simulink model "Vehicle_Model_999_Modular"  (R2025b)
settings: Solver=ode23tb  StartTime=0.0  StopTime=20  MaxStep=0.001  RelTol=1e-3
values from neighbouring files (symbols this model uses):
  aero_par = struct()    [Load_aero_parameters.m]
  init_r = 0    [Run_this_first.m]
  init_vx = 0    [Run_this_first.m]
  init_vy = 0    [Run_this_first.m]
  m = Par.m    [LapSim_Endurance_final_ts_v2.m]    (also in Lap_Sim_Final_inverse.m = Par.Mass; Lapsim_Endurance_final_ts.m; New_LapSim_final_ts_v1.m = Par.Mass; Torque_vectoring_lookup_table_v3.m = 270)
  Par = struct()    [Load_vehicle_parameters.m]
  sus_par = struct()    [Load_sus_parameters.m]
  TireData = []    [Lapsim_final_for_app.m]
  V_ref = 45    [Run_this_first.m]
undefined symbols (not defined in the file or in its folder): Battery, Brake_Val, HP, Ki_data, Kp_data, Motor, steer_input, Steer_Val, Throttle_Val, vx_breakpoints
libraries: simulink x7, autolibshared x2, BatteryEstimators x1, simulink_extras x1
(part 2 of 3)

== system Vehicle_Model_999_Modular/Vehicle dynamics/Fx, Fy calculations/Slip_angle_calculation ==
  Bus Selector25 : BusSelector  OutputSignals=Longitudinal_vel
  Bus Selector26 : BusSelector  OutputSignals=Lateral_vel
  Bus Selector27 : BusSelector  OutputSignals=Yaw_rate
  Bus Selector28 : BusSelector  OutputSignals=Steer_FL
  Bus Selector29 : BusSelector  OutputSignals=Steer_FR
  Slip Angles : MATLAB Function  TreatAsAtomicUnit=on
  Subsystem : Subsystem
  Visualize Slip_angle : Subsystem
  effective_slip_angle : Outport
  wires:
  Bus Selector26/1 -> Slip Angles/2(Lateral_vel)  "<Lateral_vel>"
  Bus Selector27/1 -> Slip Angles/3(yawrate)  "<Yaw_rate>"
  [Steer_bus] -> Bus Selector29/1, Bus Selector28/1
  [chassisbus] -> Bus Selector27/1, Bus Selector26/1, Bus Selector25/1
  Bus Selector25/1 -> Slip Angles/1(Longitudinal_vel)  "<Longitudinal_vel>"
  Slip Angles/1(slip_angles) -> Subsystem/2(slip_angles)
  Bus Selector28/1 -> Slip Angles/4(Steer_FL)  "<Steer_FL>"
  Bus Selector29/1 -> Slip Angles/5(Steer_FR)  "<Steer_FR>"
  Subsystem/1(slip_ratio) -> Visualize Slip_angle/1(slip_angle), effective_slip_angle/1  "effective_slip_angle"
  [Toe_angle] -> Subsystem/1(toe)

== system Vehicle_Model_999_Modular/Vehicle dynamics/Fx, Fy calculations/Slip_ratio_calculation ==
  Bus Selector21 : BusSelector  OutputSignals=Longitudinal_vel
  Bus Selector22 : BusSelector  OutputSignals=Yaw_rate
  Bus Selector23 : BusSelector  OutputSignals=Omega
  Bus Selector24 : BusSelector  OutputSignals=Lateral_vel
  Bus Selector32 : BusSelector  OutputSignals=Steer_FL
  Bus Selector33 : BusSelector  OutputSignals=Steer_FR
  Visualize Slip_ratios : Subsystem  Commented=on
  slip ratios : MATLAB Function  TreatAsAtomicUnit=on
  slip_ratios : Outport
  wires:
  [Steer_bus] -> Bus Selector32/1, Bus Selector33/1
  Bus Selector21/1 -> slip ratios/1(Vx)  "<Longitudinal_vel>"
  Bus Selector23/1 -> slip ratios/4(Omega)  "<Omega>"
  Bus Selector32/1 -> slip ratios/5(Steer_FL)  "<Steer_FL>"
  [chassisbus] -> Bus Selector22/1, Bus Selector24/1, Bus Selector21/1
  Bus Selector22/1 -> slip ratios/3(yawrate)  "<Yaw_rate>"
  Bus Selector33/1 -> slip ratios/6(Steer_FR)  "<Steer_FR>"
  Bus Selector24/1 -> slip ratios/2(Vy)  "<Lateral_vel>"
  [Wheel_bus] -> Bus Selector23/1
  slip ratios/1(slip_ratios) -> Visualize Slip_ratios/1(slip_ratio), slip_ratios/1  "slip_ratios"

== system Vehicle_Model_999_Modular/Vehicle dynamics/Fx, Fy calculations/Tyre_relaxation ==
  Fx_ss : Inport
  Bus Selector : BusSelector  OutputSignals=Longitudinal_vel
  Integrator : Integrator
  MATLAB Function : MATLAB Function  TreatAsAtomicUnit=on
  Fx_w : Outport
  wires:
  Fx_ss/1 -> MATLAB Function/1(Fx_ss)
  MATLAB Function/1(Fx_dot) -> Integrator/1
  Integrator/1 -> Fx_w/1, MATLAB Function/2(Fx_act)
  Bus Selector/1 -> MATLAB Function/3(Vx)  "<Longitudinal_vel>"
  [chassisbus] -> Bus Selector/1

== system Vehicle_Model_999_Modular/Vehicle dynamics/Fx, Fy calculations/Visualise_Fy_B ==
  Fy_B : Inport
  MATLAB Function : MATLAB Function  TreatAsAtomicUnit=on
  Visualise Fy_B : Scope  Commented=on  NumInputPorts=4
  wires:
  Fy_B/1 -> MATLAB Function/1(Fy_tire)
  MATLAB Function/2(Fy_B_fr) -> Visualise Fy_B/2  "Fy_B_fr"
  MATLAB Function/4(Fy_B_rr) -> Visualise Fy_B/4  "Fy_B_rr"
  MATLAB Function/1(Fy_B_fl) -> Visualise Fy_B/1  "Fy_B_fl"
  MATLAB Function/3(Fy_B_rl) -> Visualise Fy_B/3  "Fy_B_rl"

== system Vehicle_Model_999_Modular/Vehicle dynamics/Fx, Fy calculations/Visualiser ==
  mz : Inport
  mu_x : Inport  Port=2
  mu_y : Inport  Port=3
  Demux : Demux
  Demux1 : Demux
  Demux2 : Demux
  Scope : Scope  NumInputPorts=4
  Scope1 : Scope  NumInputPorts=4
  Scope2 : Scope  NumInputPorts=4
  wires:
  mz/1 -> Demux/1
  Demux/1 -> Scope/1
  Demux/2 -> Scope/2
  Demux/3 -> Scope/3
  Demux/4 -> Scope/4
  Demux1/3 -> Scope1/3
  Demux1/2 -> Scope1/2
  mu_x/1 -> Demux1/1
  Demux1/1 -> Scope1/1
  Demux1/4 -> Scope1/4
  Demux2/3 -> Scope2/3
  Demux2/2 -> Scope2/2
  mu_y/1 -> Demux2/1
  Demux2/1 -> Scope2/1
  Demux2/4 -> Scope2/4

== system Vehicle_Model_999_Modular/Vehicle dynamics/Steering/Steering Kinematics ==
  Steer_Input : Inport
  Ackermann_Pct : Inport  Port=2
  Bus Creator1 : BusCreator  Inputs=2
  Steering Kinematics : MATLAB Function  TreatAsAtomicUnit=on
  To Workspace : ToWorkspace  VariableName=steer_L  SaveFormat=Timeseries  SampleTime=-1
  To Workspace1 : ToWorkspace  VariableName=steer_R  SaveFormat=Timeseries  SampleTime=-1
  Steering Angles : Outport
  wires:
  Steering Kinematics/1(Steer_FL) -> Bus Creator1/1, To Workspace/1  "Steer_FL"
  Steer_Input/1 -> Steering Kinematics/1(Steer_Input)
  Steering Kinematics/2(Steer_FR) -> Bus Creator1/2, To Workspace1/1  "Steer_FR"
  Ackermann_Pct/1 -> Steering Kinematics/2(Ackermann_Pct)
  Bus Creator1/1 -> Steering Angles/1

== system Vehicle_Model_999_Modular/Vehicle dynamics/Suspension/Camber ==
  Zs_static : Inport
  Zs : Inport  Port=2
  DynamicCamber_FromHP_Zmeters : MATLAB Function  TreatAsAtomicUnit=on
  Subsystem : Subsystem
  Subsystem1 : Subsystem  Commented=on
  Subsystem2 : Subsystem  Commented=on
  camber_angle : Outport
  wires:
  DynamicCamber_FromHP_Zmeters/1(Camber) -> camber_angle/1, Subsystem/1(Camber)
  Zs/1 -> DynamicCamber_FromHP_Zmeters/1(Zs)
  Zs_static/1 -> DynamicCamber_FromHP_Zmeters/2(Zs_static)
  DynamicCamber_FromHP_Zmeters/2(dynamic_camber_visualisation) -> Subsystem1/1(dynamic_camber)
  DynamicCamber_FromHP_Zmeters/3(static_camber_visualisation) -> Subsystem2/1(static_camber)

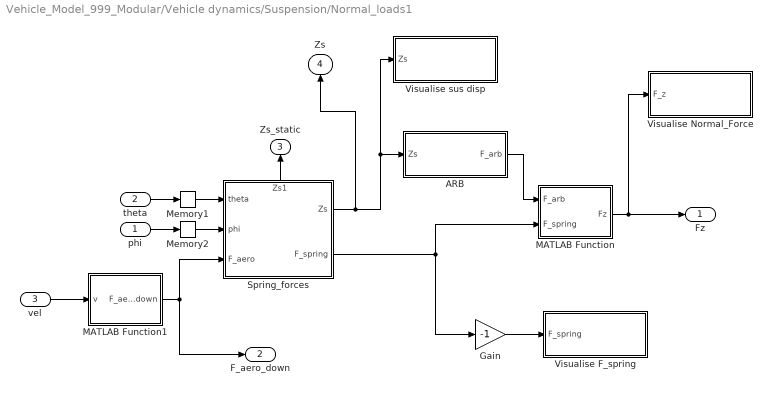
== system Vehicle_Model_999_Modular/Vehicle dynamics/Suspension/Normal_loads1 ==
  phi : Inport
  theta : Inport  Port=2
  vel : Inport  Port=3
  ARB : Subsystem
  Gain : Gain  Gain=-1
  MATLAB Function : MATLAB Function  TreatAsAtomicUnit=on
  MATLAB Function1 : MATLAB Function  TreatAsAtomicUnit=on
  Memory1 : Memory
  Memory2 : Memory
  Spring_forces : Subsystem
      settings: PortSchema="{\"entries\":[{\"content\":{\"sides\":[{\"content\":{\"connectorIds\":[\"In1\",\"In2\",\"In3\"]},\"type\":\"ConnectorPlacement.EquallySpacedRectSide\",\"uuid\":\"355bde33-3e3d-4de3-a05a-1287e2d3eebd\"},{\"content\":{\"connectorIds\":[\"Out1\",\"Out2\"],\"side\":\"RIGHT\"},\"type\":\"ConnectorPlacement.EquallySpacedRectSide\",\"uuid\":\"644c8213-6936-480f-b4bc-76ae135da058\"},{\"content\":{\"connectorIds\":[\"Out3\"],\"side\":\"TOP\"},\"type\":\"ConnectorPlacement.EquallySpacedRectSide\",\"uuid\":\"02c95e6b-ea4d-4952-978a-25b4914c2c12\"}]},\"type\":\"ConnectorPlacement.EquallySpacedConnector\",\"uuid\":\"3ff29f82-1f4c-432e-8c89-df3d4bc3a019\"}],\"packageUris\":[\"http://schema.mathworks.com/mf0/Connector/R2020b\"],\"version\":\"1.0\"}"
  Visualise F_spring : Subsystem
  Visualise Normal_Force : Subsystem
  Visualise sus disp : Subsystem
  Fz : Outport
  F_aero_down : Outport  Port=2
  Zs_static : Outport  Port=3
  Zs : Outport  Port=4
  wires:
  theta/1 -> Memory1/1
  phi/1 -> Memory2/1
  ARB/1(F_arb) -> MATLAB Function/1(F_arb)
  MATLAB Function/1(Fz) -> Visualise Normal_Force/1(F_z), Fz/1
  vel/1 -> MATLAB Function1/1(v)
  MATLAB Function1/1(F_aero_down) -> F_aero_down/1, Spring_forces/3(F_aero)
  Spring_forces/2(F_spring) -> MATLAB Function/2(F_spring), Gain/1
  Spring_forces/1(Zs) -> Visualise sus disp/1(Zs), ARB/1(Zs), Zs/1
  Spring_forces/3(Zs1) -> Zs_static/1
  Memory1/1 -> Spring_forces/1(theta)
  Memory2/1 -> Spring_forces/2(phi)
  Gain/1 -> Visualise F_spring/1(F_spring)

== system Vehicle_Model_999_Modular/Vehicle dynamics/Suspension/Toe_calculation ==
  Fy : Inport
  Fx : Inport  Port=2
  Mz : Inport  Port=3
  Mux1 : Mux
  toe_fl1 : MATLAB Function  TreatAsAtomicUnit=on
  Out2 : Outport
  wires:
  Mux1/1 -> Out2/1
  Mz/1 -> toe_fl1/3(Mz)
  Fx/1 -> toe_fl1/2(Fx_tire)
  Fy/1 -> toe_fl1/1(Fy_tire)
  toe_fl1/1(Toe_fl) -> Mux1/1
  toe_fl1/2(Toe_fr) -> Mux1/2
  toe_fl1/3(Toe_rl) -> Mux1/3
  toe_fl1/4(Toe_rr) -> Mux1/4

== system Vehicle_Model_999_Modular/Vehicle dynamics/Suspension/roll and pitch angles1 ==
  ax : Inport
  ay : Inport  Port=2
  F_aero : Inport  Port=3
  Phi_constants : MATLAB Function  TreatAsAtomicUnit=on
  Pitch : Subsystem
  Roll : Subsystem
  Scope : Scope  NumInputPorts=2
      settings: ActiveDisplayYMinimum=-1  ActiveDisplayYMaximum=1
  theta_constants : MATLAB Function  TreatAsAtomicUnit=on
  phi : Outport
  Theta : Outport  Port=2
  wires:
  ax/1 -> Pitch/3(ax)
  Phi_constants/1(K_phi) -> Roll/1(K_phi)
  Phi_constants/2(C_phi) -> Roll/2(C_phi)
  ay/1 -> Roll/3(ay)
  Roll/1(phi) -> phi/1, Scope/2
  Pitch/1(Theta) -> Scope/1, Theta/1
  theta_constants/1(K_theta) -> Pitch/1(K_theta)
  theta_constants/2(C_theta) -> Pitch/2(C_theta)
  F_aero/1 -> Pitch/4(downforce)

== system Vehicle_Model_999_Modular/Vehicle dynamics/Wheel_dynamics/Wheel Dynamics ==
  Fx_rr : Inport
  Bus Selector8 : BusSelector  OutputSignals=Fx_tyre
  Integrator : Integrator  InitialCondition=init_vx/Par.R0  LimitOutput=on  UpperSaturationLimit=1e6
  MATLAB Function : MATLAB Function  TreatAsAtomicUnit=on
  Scope : Scope
      settings: ActiveDisplayYMinimum=-1  ActiveDisplayYMaximum=1  DataLoggingVariableName=ScopeData3
  Omega : Outport
  wires:
  [Torque_inputs] -> MATLAB Function/1(T_in)
  Fx_rr/1 -> MATLAB Function/2(Fx_rr)
  MATLAB Function/1(Omega_dot) -> Integrator/1
  [Force_bus] -> Bus Selector8/1
  Bus Selector8/1 -> MATLAB Function/3(Fx_tire)  "<Fx_tyre>"
  Integrator/1 -> Scope/1, Omega/1, MATLAB Function/4(Omega)

== system Vehicle_Model_999_Modular/E-powertrain/Torque Distribution/Torque Vectoring/Target yaw rate ==
  steering angle : Inport
  Fz_4x1 : Inport  Port=2
  Dy : Inport  Port=3
  vx : Inport  Port=4
  MATLAB Function : MATLAB Function  TreatAsAtomicUnit=on
  target yaw rate : Outport
  ideal_yaw : Outport  Port=2
  wires:
  vx/1 -> MATLAB Function/1(vx)
  Fz_4x1/1 -> MATLAB Function/4(Fz)
  Dy/1 -> MATLAB Function/3(Dy)
  steering angle/1 -> MATLAB Function/2(delta)
  MATLAB Function/1(target_yaw) -> target yaw rate/1
  MATLAB Function/2(ideal_yaw) -> ideal_yaw/1

== system Vehicle_Model_999_Modular/Inputs/Brake_input_selector/Brake Variant Subsystem/GGV ==
  Constant : Constant  Value=Brake_Val
  brake_input : Outport
  wires:
  Constant/1 -> brake_input/1

== system Vehicle_Model_999_Modular/Inputs/Brake_input_selector/Brake Variant Subsystem/Sideslip_vs_curvature_cst_accln ==
  vel : Inport
  Constant : Constant  Value=10
  Constant3 : Constant  Value=0
  Longitudinal Driver : autolibshared/Longitudinal Driver  extAccelOvr=off  extDecelOvr=off  extAccelHld=off  extDecelHld=off  extAccelZero=off  extDecelZero=off  cntrlType=PI  shftType=None  velUnits=m/s  gearOut=off  Kp=10  Ki=5  Kff=.1  Kg=0  VehVelVec=[0 100]  KffVec=[.1 .1]  KpVec=[10 10]  KiVec=[5 5]  KgVec=[0 0]  m=1500  Kpt=3000  tau=.1  L=2  aR=200  bR=2.5  cR=.5  g=9.81  vnom=5  Kaw=1  tauerr=.01  tauPt=2  GearInit=0  tShift=.1  pdlVec=[0.1 0.4 0.5 0.9]  upShftTbl=[-1 12.9375 26.4375 39.9375 51.18749999999999 62.4375 72.84375 83.25;-1 16.3125 29.8125 43.3125 54.5624 65.8125 76.78125 87.75;-1 19.6875 33.1875 46.68749999999999 57.9375 69.1875 80.71875 92.25;-1 33 52.5 77.25 100.5 138.75 161.875 185]  dwnShftTbl=[1 9.5625 23.0625 36.5625 47.8125 59.0625 68.90625 78.75;1 12.9375 26.4375 39.9375 51.18749999999999 62.4375 72.84375 83.25;1 16.3125 29.8125 43.3125 54.562499 65.8125 76.78125 87.75;1 19.6875 33.1875 46.68749999999999 57.9375 69.1875 80.71875 92.25]  tClutch=.5  tRev=.5  tPark=120  aMode=2  UpGearVec="[0  1  2  3  4  5  6  7]"  DownGearVec="[1  2  3  4  5  6  7  8]"
      settings: LibrarySourceBlock=vehdynlibdriver/Longitudinal Driver
  Terminator1 : Terminator
  brake_input : Outport
  accln : Outport  Port=2
  wires:
  Constant3/1 -> Longitudinal Driver/3
  Constant/1 -> Longitudinal Driver/1
  Longitudinal Driver/1 -> Terminator1/1
  Longitudinal Driver/2 -> accln/1
  Longitudinal Driver/3 -> brake_input/1
  vel/1 -> Longitudinal Driver/2

== system Vehicle_Model_999_Modular/Inputs/Brake_input_selector/Brake Variant Subsystem/Simulink ==
  brake_sim : Inport
  brake_input : Outport
  wires:
  brake_sim/1 -> brake_input/1

== system Vehicle_Model_999_Modular/Inputs/Brake_input_selector/Brake Variant Subsystem/curvature vs steer_angle ==
  vel : Inport
  Constant : Constant  Value=V_ref
  Constant3 : Constant  Value=0
  Longitudinal Driver : autolibshared/Longitudinal Driver  extAccelOvr=off  extDecelOvr=off  extAccelHld=off  extDecelHld=off  extAccelZero=off  extDecelZero=off  cntrlType=PI  shftType=None  velUnits=m/s  gearOut=off  Kp=10  Ki=5  Kff=.1  Kg=0  VehVelVec=[0 100]  KffVec=[.1 .1]  KpVec=[10 10]  KiVec=[5 5]  KgVec=[0 0]  m=1500  Kpt=3000  tau=.1  L=2  aR=200  bR=2.5  cR=.5  g=9.81  vnom=5  Kaw=1  tauerr=.01  tauPt=2  GearInit=0  tShift=.1  pdlVec=[0.1 0.4 0.5 0.9]  upShftTbl=[-1 12.9375 26.4375 39.9375 51.18749999999999 62.4375 72.84375 83.25;-1 16.3125 29.8125 43.3125 54.5624 65.8125 76.78125 87.75;-1 19.6875 33.1875 46.68749999999999 57.9375 69.1875 80.71875 92.25;-1 33 52.5 77.25 100.5 138.75 161.875 185]  dwnShftTbl=[1 9.5625 23.0625 36.5625 47.8125 59.0625 68.90625 78.75;1 12.9375 26.4375 39.9375 51.18749999999999 62.4375 72.84375 83.25;1 16.3125 29.8125 43.3125 54.562499 65.8125 76.78125 87.75;1 19.6875 33.1875 46.68749999999999 57.9375 69.1875 80.71875 92.25]  tClutch=.5  tRev=.5  tPark=120  aMode=2  UpGearVec="[0  1  2  3  4  5  6  7]"  DownGearVec="[1  2  3  4  5  6  7  8]"
      settings: LibrarySourceBlock=vehdynlibdriver/Longitudinal Driver
  Terminator : Terminator
  brake_input : Outport
  accln : Outport  Port=2
  wires:
  Longitudinal Driver/3 -> brake_input/1
  Constant3/1 -> Longitudinal Driver/3
  Longitudinal Driver/1 -> Terminator/1
  Constant/1 -> Longitudinal Driver/1
  Longitudinal Driver/2 -> accln/1
  vel/1 -> Longitudinal Driver/2

== system Vehicle_Model_999_Modular/Inputs/Brake_input_selector/Brake Variant Subsystem/sideslip_vs_curvature ==
  brake_sim : Inport
  brake_input : Outport
  wires:
  brake_sim/1 -> brake_input/1

== system Vehicle_Model_999_Modular/Inputs/Brake_input_selector/Brake Variant Subsystem/steerdiff_vs_ay ==
  Constant : Constant  Value=0
  brake_input : Outport
  wires:
  Constant/1 -> brake_input/1

== system Vehicle_Model_999_Modular/Inputs/Brake_input_selector/Brake Variant Subsystem/timeseries ==
  From Workspace : FromWorkspace  VariableName=brake_ts
  brake_input : Outport
  wires:
  From Workspace/1 -> brake_input/1

== system Vehicle_Model_999_Modular/Inputs/Throttle_input_selector/Throttle Variant Subsystem/GGV ==
  SimInput_Throttle : Constant  Value=Throttle_Val
  throttle : Outport
  wires:
  SimInput_Throttle/1 -> throttle/1

== system Vehicle_Model_999_Modular/Inputs/Throttle_input_selector/Throttle Variant Subsystem/Simulink ==
  accln : Inport
  throttle : Outport
  wires:
  accln/1 -> throttle/1

== system Vehicle_Model_999_Modular/Inputs/Throttle_input_selector/Throttle Variant Subsystem/Timeseries ==
  From Workspace : FromWorkspace  VariableName=throttle_ts
  throttle : Outport
  wires:
  From Workspace/1 -> throttle/1

== system Vehicle_Model_999_Modular/Inputs/Throttle_input_selector/Throttle Variant Subsystem/curvature vs steer ==
  accln_input_for_map1 : Inport
  throttle : Outport
  wires:
  accln_input_for_map1/1 -> throttle/1

== system Vehicle_Model_999_Modular/Inputs/Throttle_input_selector/Throttle Variant Subsystem/sideslip_vs_curvature ==
  Constant : Constant
  throttle : Outport
  wires:
  Constant/1 -> throttle/1

== system Vehicle_Model_999_Modular/Inputs/Throttle_input_selector/Throttle Variant Subsystem/sideslip_vs_curvature_cst_accln ==
  accln_input_for_map1 : Inport
  throttle : Outport
  wires:
  accln_input_for_map1/1 -> throttle/1

== system Vehicle_Model_999_Modular/Inputs/Throttle_input_selector/Throttle Variant Subsystem/steerdiff_vs_ay ==
  Clock : Clock
  Constant1 : Constant  Value=0.25
  Ramp : simulink/Sources/Ramp  slope=2  start=0  InitialOutput=0
  Saturation : Saturate  UpperLimit=1  LowerLimit=0
  Switch : Switch  Criteria=u2 > Threshold  Threshold=4  SaturateOnIntegerOverflow=off  InputSameDT=off
  throttle : Outport
  wires:
  Clock/1 -> Switch/2
  Ramp/1 -> Switch/3
  Switch/1 -> Saturation/1
  Constant1/1 -> Switch/1
  Saturation/1 -> throttle/1

== system Vehicle_Model_999_Modular/Inputs/steer_input_selector/Steering Variant Subsystem/GGV ==
  SimInput_Steer : Constant  Value=Steer_Val
  Steer Input : Outport
  wires:
  SimInput_Steer/1 -> Steer Input/1

== system Vehicle_Model_999_Modular/Inputs/steer_input_selector/Steering Variant Subsystem/Simulink ==
  In1 : Inport
  Steer Input : Outport
  wires:
  In1/1 -> Steer Input/1

== system Vehicle_Model_999_Modular/Inputs/steer_input_selector/Steering Variant Subsystem/Timeseries ==
  From Workspace : FromWorkspace  VariableName=steer_ts
  Steer Input : Outport
  wires:
  From Workspace/1 -> Steer Input/1

== system Vehicle_Model_999_Modular/Inputs/steer_input_selector/Steering Variant Subsystem/curvature_vs_steering_angle ==
  Clock1 : Clock
  Constant1 : Constant  Value=0
  Ramp2 : simulink/Sources/Ramp  slope=pi/60  start=10  InitialOutput=0
  Saturation1 : Saturate  UpperLimit=pi/6
  Switch1 : Switch  Criteria=u2 > Threshold  Threshold=10  SaturateOnIntegerOverflow=off  InputSameDT=off
  Steer Input : Outport
  wires:
  Switch1/1 -> Saturation1/1
  Ramp2/1 -> Switch1/1
  Clock1/1 -> Switch1/2
  Constant1/1 -> Switch1/3
  Saturation1/1 -> Steer Input/1

== system Vehicle_Model_999_Modular/Inputs/steer_input_selector/Steering Variant Subsystem/sideslip_vs_curvature_1 ==
  Clock : Clock
  Constant : Constant  Value=0
  Constant1 : Constant  Value=steer_input
  Saturation : Saturate  UpperLimit=pi/20
  Switch : Switch  Criteria=u2 > Threshold  Threshold=4  SaturateOnIntegerOverflow=off  InputSameDT=off
  Steer Input : Outport
  wires:
  Switch/1 -> Saturation/1
  Saturation/1 -> Steer Input/1
  Constant1/1 -> Switch/1
  Clock/1 -> Switch/2
  Constant/1 -> Switch/3

== system Vehicle_Model_999_Modular/Inputs/steer_input_selector/Steering Variant Subsystem/sideslip_vs_curvature_constant_lat_accln ==
  Clock : Clock
  Constant : Constant  Value=0
  Ramp : simulink/Sources/Ramp  slope=pi/100  start=4  InitialOutput=0
  Saturation : Saturate  UpperLimit=pi/20
  Switch : Switch  Criteria=u2 > Threshold  Threshold=4  SaturateOnIntegerOverflow=off  InputSameDT=off
  Steer Input : Outport
  wires:
  Switch/1 -> Saturation/1
  Saturation/1 -> Steer Input/1
  Ramp/1 -> Switch/1
  Clock/1 -> Switch/2
  Constant/1 -> Switch/3

== system Vehicle_Model_999_Modular/Inputs/steer_input_selector/Steering Variant Subsystem/steerdiff_vs_ay ==
  Clock : Clock
  Constant : Constant  Value=0
  Ramp : simulink/Sources/Ramp  slope=pi/30  start=5  InitialOutput=0
  Saturation : Saturate  UpperLimit=pi/6  LowerLimit=0
  Switch : Switch  Criteria=u2 > Threshold  Threshold=5  SaturateOnIntegerOverflow=off  InputSameDT=off
  Steer Input : Outport
  wires:
  Switch/1 -> Saturation/1
  Ramp/1 -> Switch/1
  Constant/1 -> Switch/3
  Clock/1 -> Switch/2
  Saturation/1 -> Steer Input/1

== system Vehicle_Model_999_Modular/Vehicle dynamics/Force and Torque Equilibrium/Subsystem/Triggered Subsystem ==
  In1 : Inport
  Trigger : TriggerPort  VariantControl=(inherit)
  Out1 : Outport
  wires:
  In1/1 -> Out1/1

== system Vehicle_Model_999_Modular/Vehicle dynamics/Fx, Fy calculations/Slip_angle_calculation/Subsystem ==
  toe : Inport
  slip_angles : Inport  Port=2
  Subtract : Sum  Inputs=+-
  slip_ratio : Outport
  wires:
  slip_angles/1 -> Subtract/1
  toe/1 -> Subtract/2
  Subtract/1 -> slip_ratio/1

== system Vehicle_Model_999_Modular/Vehicle dynamics/Fx, Fy calculations/Slip_angle_calculation/Visualize Slip_angle ==
  slip_angle : Inport
  Demux : Demux
  To Workspace : ToWorkspace  VariableName=slip_angle_fl  SaveFormat=Timeseries  SampleTime=-1
  To Workspace1 : ToWorkspace  VariableName=slip_angle_fr  SaveFormat=Timeseries  SampleTime=-1
  To Workspace2 : ToWorkspace  VariableName=slip_angle_rl  SaveFormat=Timeseries  SampleTime=-1
  To Workspace3 : ToWorkspace  VariableName=slip_angle_rr  SaveFormat=Timeseries  SampleTime=-1
  Visualize_slip_angle : Scope  NumInputPorts=4
      settings: ActiveDisplayYMinimum=-0.21602622026058244  ActiveDisplayYMaximum=0.44480179601811975  DataLoggingVariableName=ScopeData2
  wires:
  slip_angle/1 -> Demux/1
  Demux/1 -> To Workspace/1, Visualize_slip_angle/1  "slip_angle_fl"
  Demux/2 -> To Workspace1/1, Visualize_slip_angle/2  "slip_angle_fr"
  Demux/3 -> To Workspace2/1, Visualize_slip_angle/3  "slip_angle_rl"
  Demux/4 -> To Workspace3/1, Visualize_slip_angle/4  "slip_angle_rr"

== system Vehicle_Model_999_Modular/Vehicle dynamics/Fx, Fy calculations/Slip_ratio_calculation/Visualize Slip_ratios ==
  slip_ratio : Inport
  Demux : Demux
  To Workspace : ToWorkspace  VariableName=slip_ratio_fl  SaveFormat=Timeseries  SampleTime=-1
  To Workspace1 : ToWorkspace  VariableName=slip_ratio_fr  SaveFormat=Timeseries  SampleTime=-1
  To Workspace2 : ToWorkspace  VariableName=slip_ratio_rl  SaveFormat=Timeseries  SampleTime=-1
  To Workspace3 : ToWorkspace  VariableName=slip_ratio_rr  SaveFormat=Timeseries  SampleTime=-1
  Visualize_slip_ratio : Scope  NumInputPorts=4
      settings: ActiveDisplayYMinimum=-0.089517062786901649  ActiveDisplayYMaximum=0.2451885663654759  DataLoggingVariableName=ScopeData2
  wires:
  slip_ratio/1 -> Demux/1
  Demux/1 -> To Workspace/1, Visualize_slip_ratio/1  "slip_ratio_fl"
  Demux/2 -> Visualize_slip_ratio/2, To Workspace1/1  "slip_ratio_fr"
  Demux/3 -> Visualize_slip_ratio/3, To Workspace2/1  "slip_ratio_rl"
  Demux/4 -> Visualize_slip_ratio/4, To Workspace3/1  "slip_ratio_rr"

== system Vehicle_Model_999_Modular/Vehicle dynamics/Suspension/Camber/Subsystem ==
  Camber : Inport
  Demux1 : Demux
  Gain : Gain  Gain=180/pi
  Scope : Scope  NumInputPorts=4
      settings: ActiveDisplayYMinimum=-0.50156  ActiveDisplayYMaximum=0.49315  DataLoggingVariableName=ScopeData17
  wires:
  Gain/1 -> Demux1/1
  Demux1/4 -> Scope/4  "RR"
  Demux1/3 -> Scope/3  "RL"
  Demux1/2 -> Scope/2  "FR"
  Demux1/1 -> Scope/1  "FL"
  Camber/1 -> Gain/1

== system Vehicle_Model_999_Modular/Vehicle dynamics/Suspension/Camber/Subsystem1 ==
  dynamic_camber : Inport
  Demux1 : Demux
  Gain : Gain  Gain=180/pi
  Scope : Scope  NumInputPorts=4
      settings: ActiveDisplayYMinimum=78.6694  ActiveDisplayYMaximum=79.6641  DataLoggingVariableName=ScopeData17
  wires:
  Gain/1 -> Demux1/1
  Demux1/4 -> Scope/4
  Demux1/3 -> Scope/3
  Demux1/2 -> Scope/2
  Demux1/1 -> Scope/1
  dynamic_camber/1 -> Gain/1

== system Vehicle_Model_999_Modular/Vehicle dynamics/Suspension/Camber/Subsystem2 ==
  static_camber : Inport
  Demux1 : Demux
  Gain : Gain  Gain=180/pi
  Scope : Scope  NumInputPorts=4
      settings: ActiveDisplayYMinimum=-1  ActiveDisplayYMaximum=1  DataLoggingVariableName=ScopeData17
  wires:
  static_camber/1 -> Gain/1
  Demux1/1 -> Scope/1
  Demux1/2 -> Scope/2
  Demux1/3 -> Scope/3
  Demux1/4 -> Scope/4
  Gain/1 -> Demux1/1

== system Vehicle_Model_999_Modular/Vehicle dynamics/Suspension/Normal_loads1/ARB ==
  Zs : Inport
  MATLAB Function : MATLAB Function  TreatAsAtomicUnit=on
  Visualise F_arb : Subsystem
  F_arb : Outport
  wires:
  Zs/1 -> MATLAB Function/1(Zs)
  MATLAB Function/1(F_arb) -> Visualise F_arb/1(F_arb), F_arb/1

== system Vehicle_Model_999_Modular/Vehicle dynamics/Suspension/Normal_loads1/Spring_forces ==
  theta : Inport
  phi : Inport  Port=2
  F_aero : Inport  Port=3
  MATLAB Function : MATLAB Function  TreatAsAtomicUnit=on
  Zs : Outport
  F_spring : Outport  Port=2
  Zs1 : Outport  Port=3
  wires:
  theta/1 -> MATLAB Function/1(theta)
  phi/1 -> MATLAB Function/2(phi)
  F_aero/1 -> MATLAB Function/3(F_aero_total)
  MATLAB Function/2(F_spring) -> F_spring/1
  MATLAB Function/1(Zs) -> Zs/1
  MATLAB Function/3(Zs1) -> Zs1/1

== system Vehicle_Model_999_Modular/Vehicle dynamics/Suspension/Normal_loads1/Visualise F_spring ==
  F_spring : Inport
  Demux : Demux
  Scope : Scope  NumInputPorts=4
      settings: ActiveDisplayYMinimum=480.58792478811586  ActiveDisplayYMaximum=525.6458571446484  DataLoggingVariableName=ScopeData26
  wires:
  Demux/1 -> Scope/1  "F_s_fl"
  Demux/2 -> Scope/2  "F_s_fr"
  Demux/3 -> Scope/3  "F_s_rl"
  Demux/4 -> Scope/4  "F_s_rr"
  F_spring/1 -> Demux/1

== system Vehicle_Model_999_Modular/Vehicle dynamics/Suspension/Normal_loads1/Visualise Normal_Force ==
  F_z : Inport
  Demux : Demux
  Scope : Scope  NumInputPorts=4
      settings: ActiveDisplayYMinimum=596.18923674793643  ActiveDisplayYMaximum=660.49565359824726  DataLoggingVariableName=ScopeData26
  wires:
  Demux/4 -> Scope/4  "Fz_rr"
  Demux/3 -> Scope/3  "Fz_rl"
  Demux/2 -> Scope/2  "Fz_fr"
  Demux/1 -> Scope/1  "Fz_fl"
  F_z/1 -> Demux/1

== system Vehicle_Model_999_Modular/Vehicle dynamics/Suspension/Normal_loads1/Visualise sus disp ==
  Zs : Inport
  Gain : Gain  Gain=-1000
  To Workspace : ToWorkspace  VariableName=FL_wheel_displacement  SaveFormat=Timeseries  SampleTime=-1
  To Workspace1 : ToWorkspace  VariableName=FR_wheel_displacement  SaveFormat=Timeseries  SampleTime=-1
  To Workspace2 : ToWorkspace  VariableName=RL_wheel_displacement  SaveFormat=Timeseries  SampleTime=-1
  To Workspace3 : ToWorkspace  VariableName=RR_wheel_displacement  SaveFormat=Timeseries  SampleTime=-1
  Zs in mm : MATLAB Function  TreatAsAtomicUnit=on
  Zs_in mm : Scope  NumInputPorts=4
      settings: ActiveDisplayYMinimum=-1  ActiveDisplayYMaximum=1  DataLoggingVariableName=ScopeData26
  wires:
  Zs/1 -> Gain/1
  Zs in mm/1(zsfl) -> Zs_in mm/1, To Workspace/1  "zsfl in mm"
  Zs in mm/2(zsfr) -> To Workspace1/1, Zs_in mm/2  "zsfr in mm"
  Zs in mm/3(zsrl) -> To Workspace2/1, Zs_in mm/3  "zsrl  in mm"
  Zs in mm/4(zsrr) -> To Workspace3/1, Zs_in mm/4  "zsrr in mm"
  Gain/1 -> Zs in mm/1(Zs)

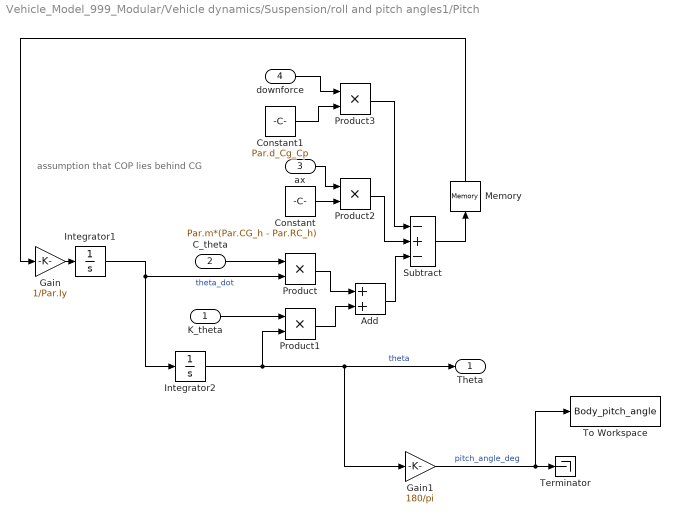
== system Vehicle_Model_999_Modular/Vehicle dynamics/Suspension/roll and pitch angles1/Pitch ==
  note: assumption that COP lies behind CG
  K_theta : Inport
  C_theta : Inport  Port=2
  ax : Inport  Port=3
  downforce : Inport  Port=4
  Add : Sum
  Constant : Constant  Value=Par.m*(Par.CG_h - Par.RC_h)
  Constant1 : Constant  Value=Par.d_Cg_Cp
  Gain : Gain  Gain=1/Par.Iy
  Gain1 : Gain  Gain=180/pi
  Integrator1 : Integrator
  Integrator2 : Integrator
  Memory : Memory
  Product{,1..3} (4 alike) : Product
  Subtract : Sum  Inputs=-+-
  Terminator : Terminator
  To Workspace : ToWorkspace  VariableName=Body_pitch_angle  SaveFormat=Timeseries  SampleTime=-1
  Theta : Outport
  wires:
  Gain/1 -> Integrator1/1
  Integrator1/1 -> Product/2, Integrator2/1  "theta_dot"
  C_theta/1 -> Product/1
  Integrator2/1 -> Theta/1, Gain1/1, Product1/2  "theta"
  K_theta/1 -> Product1/1
  Product/1 -> Add/1
  Product1/1 -> Add/2
  ax/1 -> Product2/1
  Constant/1 -> Product2/2
  Product2/1 -> Subtract/2
  Add/1 -> Subtract/3
  Subtract/1 -> Memory/1
  Memory/1 -> Gain/1
  downforce/1 -> Product3/1
  Constant1/1 -> Product3/2
  Product3/1 -> Subtract/1
  Gain1/1 -> To Workspace/1, Terminator/1  "pitch_angle_deg"

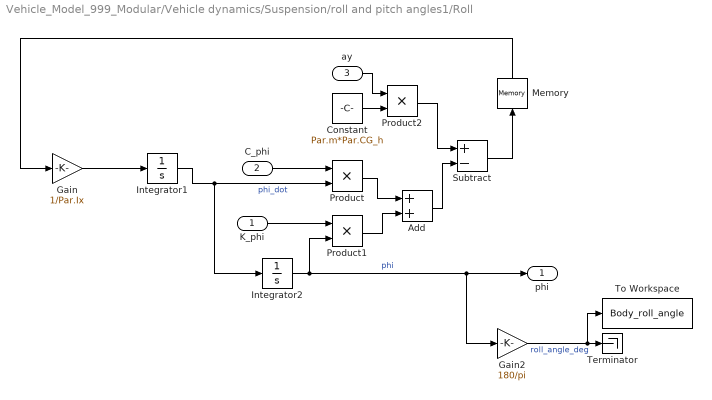
== system Vehicle_Model_999_Modular/Vehicle dynamics/Suspension/roll and pitch angles1/Roll ==
  K_phi : Inport
  C_phi : Inport  Port=2
  ay : Inport  Port=3
  Add : Sum
  Constant : Constant  Value=Par.m*Par.CG_h
  Gain : Gain  Gain=1/Par.Ix
  Gain2 : Gain  Gain=180/pi
  Integrator1 : Integrator
  Integrator2 : Integrator
  Memory : Memory
  Product : Product
  Product1 : Product
  Product2 : Product
  Subtract : Sum  Inputs=+-
  Terminator : Terminator
  To Workspace : ToWorkspace  VariableName=Body_roll_angle  SaveFormat=Timeseries  SampleTime=-1
  phi : Outport
  wires:
  Subtract/1 -> Memory/1
  Add/1 -> Subtract/2
  Product2/1 -> Subtract/1
  Constant/1 -> Product2/2
  ay/1 -> Product2/1
  Product1/1 -> Add/2
  Product/1 -> Add/1
  K_phi/1 -> Product1/1
  Integrator2/1 -> Gain2/1, phi/1, Product1/2  "phi"
  C_phi/1 -> Product/1
  Integrator1/1 -> Integrator2/1, Product/2  "phi_dot"
  Gain/1 -> Integrator1/1
  Memory/1 -> Gain/1
  Gain2/1 -> To Workspace/1, Terminator/1  "roll_angle_deg"

== system Vehicle_Model_999_Modular/Vehicle dynamics/Suspension/Normal_loads1/ARB/Visualise F_arb ==
  F_arb : Inport
  Demux : Demux
  Scope : Scope  NumInputPorts=4
      settings: ActiveDisplayYMinimum=-1  ActiveDisplayYMaximum=1  DataLoggingVariableName=ScopeData11
  wires:
  F_arb/1 -> Demux/1
  Demux/1 -> Scope/1  "F_arb_fl"
  Demux/2 -> Scope/2  "F_arb_fr"
  Demux/3 -> Scope/3  "F_arb_rl"
  Demux/4 -> Scope/4  "F_arb_rr"

== matlab function Vehicle_Model_999_Modular/Vehicle dynamics/Fx, Fy calculations/Wheel to Vehicle Coordinates ==
  data: Fx_w input; Fx_b output; Fy_w input; Steer_FL input; Steer_FR input; Fy_b output
function [Fx_b, Fy_b] = fcn(Fx_w, Fy_w, Steer_FL, Steer_FR)
%#codegen
% FORCE & MOMENT RESOLVER

    % 0. Enforce Column Vectors (Protects against array dimension mismatch)
    Fx_w = Fx_w(:);
    Fy_w = Fy_w(:);

    % 1. Construct Steering Vector [FL; FR; RL; RR]
    % Rear steering is assumed to be 0
    Delta = [Steer_FL; Steer_FR; 0; 0];
    
    % 2. Pre-calculate Trig functions (Vectorized)
    c_d = cos(Delta);
    s_d = sin(Delta);
    
    % 3. Resolve Forces into Body Frame
    % Longitudinal Body Force:
    Fx_b = Fx_w .* c_d - Fy_w .* s_d;
    
    % Lateral Body Force:
    % Fy_body = Fx_wheel * sin(delta) + Fy_wheel * cos(delta)
    Fy_b = Fx_w .* s_d + Fy_w .* c_d;
    
    % 4. Summation: Total Forces acting on CG (Uncomment if needed as outputs)
    % B_Fx = sum(Fx_b);
    % B_Fy = sum(Fy_b);
    
end

== matlab function Vehicle_Model_999_Modular/Vehicle dynamics/Wheel_dynamics/Rolling Resistance ==
  data: Fz input; wFx_rr output; Omega input; slip_angles input; Par parameter
function wFx_rr  = fcn(Fz, Omega,slip_angles, Par)
%#codegen

    % 1. Calculate Total Magnitude
    F_mag = Par.C_rr .* abs(Fz);

    % 2. Determine Direction
    Dir = tanh(10 * Omega);

    
    % X-Component: Resists Spin (Torque generating)
    % wFx = -Magnitude * Direction * cos(Alpha)
    wFx_rr = -F_mag .*Dir.* cos(slip_angles);

end

== matlab function Vehicle_Model_999_Modular/Vehicle dynamics/Wheel_dynamics/Wheel Dynamics/MATLAB Function ==
  data: T_in input; Omega_dot output; Fx_rr input; Fx_tire input; Omega input; Par parameter; Motor parameter
function Omega_dot = fcn(T_in, Fx_rr, Fx_tire, Omega, Par,Motor)
%#codegen
    
    % 1. Enforce Column Vectors
    T_in = T_in(:);
    Fx_rr = Fx_rr(:);
    Fx_tire = Fx_tire(:);
    Omega = Omega(:);
    
    % 2. Constants
    R = Par.R0;
    Iw = Par.Iw;
    b_w = 0.1; 
    derate_coefficient = 0.99;
    % 3. Soft Rev Limiter (Torque Derating)
    % Widened window (8500 to 9000 RPM) to reduce solver stiffness
    rpm_upper = Motor.n_max * (2 * pi / 60)/Motor.gear_ratio; 
    rpm_lower = Motor.n_max*derate_coefficient * (2 * pi / 60)/Motor.gear_ratio; 
    
    % Calculate derate factor: 1 when below limit, smoothly approaches 0
    derate_factor = (rpm_upper - Omega) ./ (rpm_upper - rpm_lower);
    derate_factor = max(0, min(1, derate_factor)); 
    
    % 4. Separate Drive and Brake capacities
    % Apply derate factor ONLY to positive torque (Drive)
    T_drive = max(T_in, 0) .* derate_factor; 
    T_brake_capacity = abs(min(T_in, 0)); 
    
    % 5. Smooth directional multiplier
    % Reduced steepness from 10 to 2 to prevent micro-stepping at 0 RPM
    Rotation_Dir = tanh(2 .* Omega);
    
    % 6. Calculate external torques BEFORE brakes are applied
    T_tire_reaction = abs(Fx_rr .* R) .* Rotation_Dir;
    T_tire = Fx_tire .* R;
    T_damping = b_w .* Omega;
    
    % Net torque tending to move the wheel
    T_pre_brake = T_drive - T_tire_reaction - T_tire - T_damping;
    
    % 7. Continuous Blended Brake Logic
    T_brake_dynamic = -T_brake_capacity .* Rotation_Dir;
    T_brake_static = -max(min(T_pre_brake, T_brake_capacity), -T_brake_capacity);
    
    % Reduced steepness from 10 to 2 here as well
    moving_flag = abs(tanh(2 .* Omega));
    T_brake_actual = (moving_flag .* T_brake_dynamic) + ((1 - moving_flag) .* T_brake_static);
    
    % 8. Compute Angular Acceleration
    T_net = T_pre_brake + T_brake_actual;
    Omega_dot = T_net ./ Iw;
    
end

== matlab function Vehicle_Model_999_Modular/Vehicle dynamics/Suspension/Normal_loads1/MATLAB Function1 ==
  data: v input; F_aero_down output; aero_par parameter
function F_aero_down = fcn(v,aero_par)

% Aerodynamic constants:
rho = aero_par.rho;
area = aero_par.Area;
Cl = aero_par.Cl;

F_aero_down = -0.5*rho*Cl*area*(v^2);

== matlab function Vehicle_Model_999_Modular/E-powertrain/Torque Distribution/MATLAB Function ==
  data: T_wheel input; omega input; T_FL output; T_brake_vec input; T_FR output; T_RL output; T_RR output
function [T_FL, T_FR, T_RL, T_RR] = torque_combiner(T_wheel, omega, T_brake_vec)
%#codegen
    % INPUTS:
    % T_wheel:     4x1 [FL, FR, RL, RR] Motor Torque Request (from Throttle)
    % omega:       4x1 [FL, FR, RL, RR] Wheel Speeds (rad/s)
    % T_brake_vec: 4x1 Brake Capacity (Negative values expected)
    
    % --- 1. INITIALIZATION ---
    T_FL = 0.0; T_FR = 0.0; T_RL = 0.0; T_RR = 0.0;
    
    % PARAMETERS
    w_threshold = 2.0;  % [rad/s] Speed below which we switch to linear damping
    brake_active_threshold = 100.0; % [Nm] Torque to consider "Brakes Active"
    
    % Get absolute brake capacities
    B_FL = abs(T_brake_vec(1));
    B_FR = abs(T_brake_vec(2));
    B_RL = abs(T_brake_vec(3));
    B_RR = abs(T_brake_vec(4));
    
    % --- 2. BRAKE PRIORITY LOGIC (The Fix for Rear Spin) ---
    % If the driver is braking hard, we CUT motor torque.
    % This prevents the "fighting" that causes the rear wheels to spin at 115 rad/s.
    total_brake_force = B_FL + B_FR + B_RL + B_RR;
    
    % Factor: 1.0 = Full Drive, 0.0 = Throttle Cut
    % If braking > threshold, we cut throttle to 0.
    if total_brake_force > brake_active_threshold
        throttle_factor = 0.0; 
    else
        throttle_factor = 1.0;
    end
    
    % Apply the cut to the motor inputs
    T_motor_effective = T_wheel * throttle_factor;
    
    % --- 3. ROBUST BRAKE CALCULATION (Viscous Region) ---
    % This local logic prevents solver crashes when wheels lock (w=0)
    % It uses linear damping near zero speed.
    
    % Fronts (Motor + Brake) - Front motors evaluate to 0
    T_FL = T_motor_effective(1) + apply_brake_physics(omega(1), B_FL, w_threshold);
    T_FR = T_motor_effective(2) + apply_brake_physics(omega(2), B_FR, w_threshold);
    
    % Rears (Motor + Brake)
    T_brake_RL = apply_brake_physics(omega(3), B_RL, w_threshold);
    T_brake_RR = apply_brake_physics(omega(4), B_RR, w_threshold);
    
    % Combine: Effective Motor (Positive) + Braking (Negative)
    T_RL = T_motor_effective(3) + T_brake_RL;
    T_RR = T_motor_effective(4) + T_brake_RR;
end

% --- HELPER LOGIC ---
function T_out = apply_brake_physics(w, Capacity, w_th)
    % If moving fast: Constant Friction (Capacity)
    % If moving slow: Viscous Damping (Linear line to 0)
    if abs(w) < w_th
        % Linear region (Like moving through honey)
        % This forces the torque to exactly 0 as speed hits 0.
        T_out = -Capacity * (w / w_th);
    else
        % Sliding region (Full friction)
        T_out = -Capacity * sign(w);
    end
end

== matlab function Vehicle_Model_999_Modular/E-powertrain/Torque Distribution/Torque Vectoring/MATLAB Function ==
  data: vectored_torques output; wheel_torques input; yaw_moment input; Par parameter; Motor parameter
function vectored_torques = fcn(wheel_torques,yaw_moment,Par,Motor)
max_wheel_torque = Motor.T_peak_limit * Motor.gear_ratio* Motor.overall_efficiency;
torque_difference = yaw_moment*(Par.R0/(Par.TW));
T_FL = wheel_torques(1);    
T_FR = wheel_torques(2);
T_RL = max(0,min(wheel_torques(3) - (torque_difference/2),max_wheel_torque));
T_RR = max(0,min(wheel_torques(4) + (torque_difference/2),max_wheel_torque));

vectored_torques = [T_FL; T_FR; T_RL; T_RR];

== matlab function Vehicle_Model_999_Modular/E-powertrain/Torque Distribution/Torque Vectoring/PID controller in time domain ==
  settings: updateMethod=DISCRETE
  data: ref input; yaw_moment output; y input; Kp input; Ki input; Par parameter; u_unsat output; error output; Motor parameter
function [yaw_moment,u_unsat,error] = pid_controller(ref, y, Kp, Ki,Par,Motor)
T = Par.TW;
R0 = Par.R0;
Half_T = T/2;


% Custom PI Controller with Clamping Anti-Windup

% Motor torque limits
T_max_motor = Motor.T_peak_limit*Motor.gear_ratio*Motor.overall_efficiency;  
T_min_motor = 0;  

% Force limit of each tire:
f_max = T_max_motor/R0;
f_min = T_min_motor/R0;

% Yaw_moment limits
u_max = f_max * Half_T;
u_min = f_min * Half_T;

% Persistent variables
persistent integral prev_error;
if isempty(integral)
    integral = 0;
    prev_error = 0;
end

% Sample time
T = 0.001;

% Compute error
error = ref - y;

% **Proportional Term**
P = Kp * error;

% **Integral Term with Clamping**
I = Ki * integral;

% Compute raw control signal
u_unsat = P + I;

%Clamping Anti-Windup
if u_unsat > u_max
    yaw_moment = u_max;
    % Freeze integral
elseif u_unsat < u_min
    yaw_moment = u_min;
    % Freeze integral
else
    yaw_moment = u_unsat;
    % Update integral only if NOT saturated
    integral = integral + 0.5* T * (error + prev_error);
end

% Store previous error
prev_error = error;
end

== matlab function Vehicle_Model_999_Modular/E-powertrain/Torque Distribution/Torque Vectoring/Target yaw rate/MATLAB Function ==
  data: vx input; target_yaw output; delta input; Dy input; Fz input; Par parameter; ideal_yaw output
function  [target_yaw,ideal_yaw]= target_yaw_rate(vx,delta,Dy,Fz,Par)

    ku = (Par.Lr*Par.m/(35238.459*(Par.Lf+Par.Lr))) - (Par.Lf*Par.m/(35033.582*(Par.Lf+Par.Lr)));   %understeer gradient
    epsilon = 0.01;                                                                                 %prevent division by zero
    ideal_yaw = delta*vx/(((vx+epsilon)^2*ku)+(Par.Lf+Par.Lr));                                     %from Ackermann formula

    if delta > deg2rad(1) || delta < -deg2rad(8) && vx > 3
        
        epsilon = 0.01;                                                                             %prevent division by zero
        
        mu_4x1 = Dy./Fz;                                                                            %from tire formula
        avg_mu = mean(mu_4x1(3:4));   % RL RR (if order = [FL FR RL RR])
        mu_4x1 = avg_mu;   
        
        yaw_limit = mu_4x1*Par.g/(vx + epsilon);                                                    %accounting grip limits
        
        if ideal_yaw < - yaw_limit 
            target_yaw = - yaw_limit;
        elseif ideal_yaw > yaw_limit
            target_yaw = yaw_limit;
        else 
            target_yaw = ideal_yaw;
        end
    else
    target_yaw = 0;
    end
end

== matlab function Vehicle_Model_999_Modular/Vehicle dynamics/Suspension/Toe_calculation/toe_fl1 ==
  data: Fy_tire input size=[4 1]; Fx_tire input size=[4 1]; Toe_fl output; Mz input size=[4 1]; sus_par parameter; Toe_fr output; Toe_rl output; Toe_rr output
function [Toe_fl,Toe_fr,Toe_rl,Toe_rr] = fcn(Fy_tire,Fx_tire,Mz,sus_par)

Toe_fl = sus_par.Toe_f_static + sus_par.C_Fx_toe*Fx_tire(1) + sus_par.C_Fy_toe*Fy_tire(1) + sus_par.C_Mz_toe*Mz(1);

Toe_fr = sus_par.Toe_f_static + sus_par.C_Fx_toe*Fx_tire(2) +sus_par.C_Fy_toe*Fy_tire(2) + sus_par.C_Mz_toe*Mz(2);

Toe_rl = sus_par.Toe_f_static + sus_par.C_Fx_toe*Fx_tire(3) +sus_par.C_Fy_toe*Fy_tire(3) + sus_par.C_Mz_toe*Mz(3);

Toe_rr = sus_par.Toe_f_static + sus_par.C_Fx_toe*Fx_tire(4) +sus_par.C_Fy_toe*Fy_tire(4) + sus_par.C_Mz_toe*Mz(4);

== matlab function Vehicle_Model_999_Modular/E-powertrain/Battery Pack/MATLAB Function ==
  data: Voc_pack input; v_bus output; R0_pack input; V_rc input; I_dc input
function v_bus = fcn(Voc_pack, R0_pack, V_rc, I_dc)
    % This function calculates the terminal voltage of the battery pack.
    % Voc_pack: Output from OCV LUT multiplied by Ns
    % R0_pack:  Output from R0 LUT multiplied by (Ns/Np)
    % V_rc:     Instantaneous voltage across the RC branch
    % I_dc:     Total DC current from the motor

    % 1. Calculate the instantaneous Ohmic drop (Ohm's Law)
    V_ohmic = I_dc * R0_pack;

    % 2. Calculate terminal voltage (Vt = Voc - V_ohmic - V_rc)
    v_bus = Voc_pack - V_ohmic - V_rc;

    % 3. Safety: Ensure voltage doesn't drop below a physical floor (e.g., 2.5V * Ns)
    % This prevents simulation crashes if the battery is fully depleted.
    % v_bus = max(v_bus, 2.5 * 144); 
end

== matlab function Vehicle_Model_999_Modular/E-powertrain/Torque Distribution/Traction Control/MATLAB Function1 ==
  settings: updateMethod=DISCRETE
  data: lambda_ref input; lambda_actual input size=[4 1]; throttle_cmd output; Kp input; Ki input; Kd input
function throttle_cmd = pid_traction_controller(lambda_ref, lambda_actual, ...
Kp, Ki, Kd)
%#codegen

dt = 0.001;

persistent integrator prev_error;

if isempty(integrator)
    integrator = 0;
end

if isempty(prev_error)
    prev_error = 0;
end

    % ── Error ───────────────────────────────────────
    e = lambda_ref - lambda_actual(3);

    % ── Derivative (rate of slip change) ────────────
    de = (e - prev_error) / dt;

    % ── Conditional Integration (ANTI-WINDUP) ───────
    if abs(e) < 0.2   % integrate only near target
        integrator = integrator + e * dt;
    end

    integrator = max(min(integrator, 0.5), -0.5);

    % ── PID Output ──────────────────────────────────
    throttle_pid = Kp * e + Ki * integrator + Kd * de;

    % ── Clamp output ────────────────────────────────
    throttle_pid = max(min(throttle_pid, 1.0), 0.0);

    % ── Traction control logic ──────────────────────
    throttle_cmd = throttle_pid;

    % ── Store previous error ────────────────────────
    prev_error = e;


end

== matlab function Vehicle_Model_999_Modular/E-powertrain/Torque Distribution/Traction Control/MATLAB Function ==
  data: u input; y output
function y = fcn(u)
y = zeros(4,1);
y(3) = u;
y(4) = u;

== matlab function Vehicle_Model_999_Modular/Vehicle dynamics/Rolling and Drag forces/Aero Drag ==
  data: vx input; B_F_aero output; vy input; aero_par parameter
function B_F_aero = fcn(vx, vy, aero_par)

    %#codegen
    % AERODYNAMIC DRAG (Body Frame)
    % Calculates drag vector acting on the CG.
%
% Inputs:
%   vx, vy : Vehicle Velocities in Body Frame [m/s]
%   Par    : Parameters (.Cd, .Area, .rho, .C_side)
%
% Output:
%   B_F_aero : [Fx; Fy; 0] Aerodynamic Force Vector [N]

    % 1. Longitudinal Drag (Standard)
    % Fx = -0.5 * rho * Cd * Area * vx^2
    % Usage: sign(vx) ensures drag always opposes motion
    Fx_drag = 0.5 * aero_par.rho * aero_par.Cd * aero_par.Area * vx * abs(vx);

    % 2. Lateral Drag (Side Force) - Optional
    % Only relevant if sliding significantly.
    % If Par.C_side is not defined, calculate as 0.
    if isfield(aero_par, 'C_side') && aero_par.C_side > 0
        % Side area is often approx same as Frontal Area or larger
        % Fy = - 0.5 * rho * C_side * Area_Side * vy^2
        Fy_drag = -0.5 * aero_par.rho * aero_par.C_side * aero_par.Area * vy * abs(vy);
    else
        Fy_drag = 0;
    end
    
    % 3. Output Vector for Equilibrium Block
    B_F_aero = [Fx_drag; Fy_drag; 0];

end

== matlab function Vehicle_Model_999_Modular/Vehicle dynamics/Brakes/MATLAB Function ==
  data: brake_pedal input; T_brakes output; omega input; Brake parameter; T_mag_Front output; T_mag_Rear output
function [T_brakes,T_mag_Front,T_mag_Rear]  = fcn(brake_pedal, omega, Brake)
    % BRAKE TORQUE CALCULATION
    % Converts normalized pedal/actuator position into physical torque
    % and ensures torque direction opposes wheel rotation.
    
    % 1. Calculate Magnitude of Torque based on Command (0-1)
    % We use the static max targets from the design sheet
    T_mag_Front = brake_pedal * Brake.MaxTorque_Wheel_F;
    T_mag_Rear  = brake_pedal * Brake.MaxTorque_Wheel_R;
    
    % Initialize output vector (FL, FR, RL, RR)
    T_brakes = zeros(4, 1);
    
    % 2. Apply Torque per Wheel with Directional Logic
    % Loop through all 4 wheels to apply logic individually
    % Indices: 1=FL, 2=FR, 3=RL, 4=RR
    
    for i = 1:4
        % Determine if this is a Front (1,2) or Rear (3,4) wheel
        if i <= 2
            T_req = T_mag_Front;
        else
            T_req = T_mag_Rear;
        end
        
        % Directional Check:
        % Torque must be negative if omega is positive, and vice versa.
        % -sign(omega) flips the torque direction.
        T_applied = T_req * -sign(omega(i));
        
        % Zero-Speed Cutoff:
        % If wheel is nearly stopped, clamp torque to zero to prevent 
        % the simulation from "driving" the car backwards.
        % if abs(omega(i)) < Brake.ZeroSpeedThreshold
        %     T_applied = 0;
        % 
            % Advanced: Ideally, below threshold, T_brake should act as 
            % a viscous damper or Coulomb friction that exactly cancels 
            % remaining motion, but zeroing is sufficient for laptime sims.
        % end
        
        T_brakes(i) = T_applied;
    end
end

== matlab function Vehicle_Model_999_Modular/Vehicle dynamics/Rolling and Drag forces/MATLAB Function ==
  data: u input; y output
function y = fcn(u)

y = u(1);

== matlab function Vehicle_Model_999_Modular/Vehicle dynamics/Rolling and Drag forces/Rolling Forces ==
  data: Fz input; Fx_rr_b output; Steer_FL input; Steer_FR input; Fy_rr_b output; Par parameter
function [Fx_rr_b, Fy_rr_b] = fcn(Fz, Steer_FL, Steer_FR, Par)

    %#codegen

    % 1. Setup
    C_rr = Par.C_rr; 
    
    % Construct Steering Vector (Assuming Rear Steer = 0)
    Delta = [Steer_FL; Steer_FR; 0; 0];

    % Initialize Outputs
    Fx_rr_b = zeros(4, 1);
    Fy_rr_b = zeros(4, 1);

    % 2. Calculate & Resolve Forces (Vectorized Loop)
    for i = 1:4
        
        % Magnitude (Always positive Fz)
        F_mag = C_rr * abs(Fz(i));
        
        % B. Define Force Vector in Wheel Frame
        F_xw = - F_mag;
        F_yw = 0;
        
        % C. Transform to Body Frame (Rotation)
        d = Delta(i);
        c = cos(d);
        s = sin(d);
        
        % Rotate: F_body = Rz(delta) * F_wheel
        % Fx_b = Fx_w*cos - Fy_w*sin
        Fx_rr_b(i) = F_xw * c - F_yw * s;
        
        % Fy_b = Fx_w*sin + Fy_w*cos
        Fy_rr_b(i) = F_xw * s + F_yw * c;
    end

end

== matlab function Vehicle_Model_999_Modular/Vehicle dynamics/Force and Torque Equilibrium/Force and Torque Equilibrium ==
  data: B_Fx input; ax output size=1; ay output size=1; B_Fy input; B_Fx_roll input; B_Fy_roll input; B_F_drag input; yawrate input; vx input; vy input; r_dot output size=1; Par parameter; ay_sensor output; ax_sensor output
function [ax, ay, r_dot, ay_sensor, ax_sensor] = fcn(B_Fx, B_Fy, B_Fx_roll, B_Fy_roll, B_F_drag, yawrate, vx, vy, Par)
%#codegen

    % 1. Enforce Column Vectors 
    % (Protects against dimension mismatch if an input is accidentally 1x4)
    B_Fx = B_Fx(:);
    B_Fy = B_Fy(:);
    B_Fx_roll = B_Fx_roll(:);
    B_Fy_roll = B_Fy_roll(:);
    
    % 2. Geometry Setup
    m = Par.m;
    Iz = Par.Iz;
    
    % Create Geometry Vectors for [FL; FR; RL; RR]
    % x_arms: Distance from CG to axle (Positive = Front)
    x_arms = [Par.Lf;   Par.Lf;  -Par.Lr;  -Par.Lr];
    
    % y_arms: Distance from centerline (Positive = Left)
    t = Par.TW / 2;
    y_arms = [ t;      -t;        t;      -t];
    
    % 3. Total Corner Forces
    Fx_total = B_Fx + B_Fx_roll; 
    Fy_total = B_Fy + B_Fy_roll; 
    
    % 4. Linear Force Equilibrium
    Sigma_Fx = sum(Fx_total) - B_F_drag(1);
    Sigma_Fy = sum(Fy_total) - B_F_drag(2);
    
    % 5. Linear Accelerations 
    ax = (Sigma_Fx / m) + (vy * yawrate);
    ay = (Sigma_Fy / m) - (vx * yawrate);
    
    ax_sensor = Sigma_Fx / m;
    ay_sensor = Sigma_Fy / m;
    
    % 6. Moment Equilibrium (Vectorized)
    Mz_individual = (x_arms .* Fy_total) - (y_arms .* Fx_total);
    Sigma_Mz = sum(Mz_individual);
    
    % 7. Yaw Acceleration (rad/s^2)
    r_dot = Sigma_Mz / Iz;
end

== matlab function Vehicle_Model_999_Modular/E-powertrain/Torque Distribution/Traction Control/MATLAB Function2 ==
  data: TC_output output; torque_pid input; torque_wheel input
function TC_output = fcn(torque_pid, torque_wheel)
% Initialize TC_output
TC_output = zeros(4,1);

for i = 1:4

    if torque_pid(i) < torque_wheel(i)
        TC_output(i) = torque_pid(i);
    else
        TC_output(i) = torque_wheel(i);
    end
end
